simulink model "Speedgoat_FXLMS_ANC_model"  (R2022a)
settings: Solver=FixedStepDiscrete  StartTime=0.0  StopTime=inf  RelTol=1e-3
InitFcn:
  | L = 512;
  | FS = 8000;
  | %[noise,FS] = audioread('washing8kmod.wav');
StopFcn:
  | %postCallback;
undefined symbols (not defined in the file or in its folder): Ended, Single
libraries: speedgoatlib_IO104 x3, simulink x3, dspadpt3 x3, dspsrcs4 x2, slrealtimeobsoletelib x2, audiomeasurements x1
settings Model: SimulationMode=external  Creator=The MathWorks, Inc.  LastModifiedBy=Administrator
settings SolverCC: ConcurrentTasks=on  AlgebraicLoopSolver=TrustRegion  AutoInsertRateTranBlk=on  InsertRTBMode=Never (minimum delay)
settings DataIOCC: SaveFormat=StructureWithTime  ReturnWorkspaceOutputs=off
settings OptimizationCC: BlockReduction=off  OptimizeBlockIOStorage=off  BufferReuse=off  GlobalBufferReuse=off  ExpressionFolding=off  LocalBlockOutputs=off  OptimizeDataStoreBuffers=off  BusAssignmentInplaceUpdate=off
settings DebuggingCC: UnconnectedInputMsg=warning  UnconnectedOutputMsg=warning  UnconnectedLineMsg=warning  SFExecutionAtInitializationDiag=none  SFMachineParentedDataDiag=warning  ArithmeticOperatorsInVariantConditions=warning
settings HardwareCC: ProdBitPerPointer=32  ProdBitPerSizeT=32  ProdBitPerPtrDiffT=32  ProdLargestAtomicFloat=None  ProdWordSize=32  ProdLongLongMode=on  ProdHWDeviceType=Generic->32-bit x86 compatible
settings SFSimCC: SimUseLocalCustomCode=off  CustomCodeUndefinedFunction=UseInterfaceOnly
settings RTWCC: Description=Simulink Real-Time  SystemTargetFile=slrt.tlc  TLCOptions=-axPCMaxOverloads=10000 -axPCOverLoadLen=200  TemplateMakefile=slrt_default_tmf  RTWUseLocalCustomCode=off  RTWCompilerOptimization=on
settings CodeAppCC: StateflowObjectComments=on
settings SimulinkRealTimeCC: SupportVariableSizeSignals=on  OptimizeReductions=off  RL32LogTETModifier=off  RL32LogBufSizeModifier=100e6  RL32IRQSourceModifier=Auto (PCI only)  xPCConcurrentTasks=on

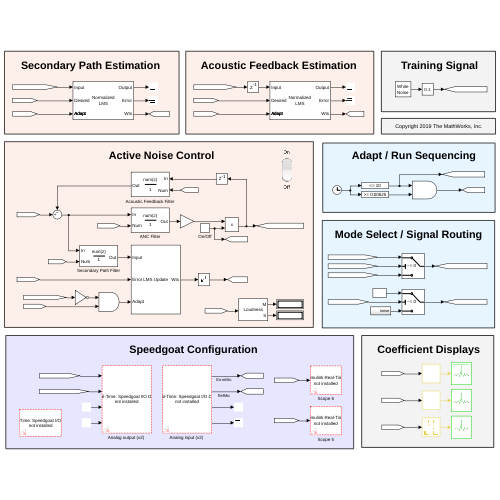
[thumbnail: Simulink's stored preview of the top-level diagram]
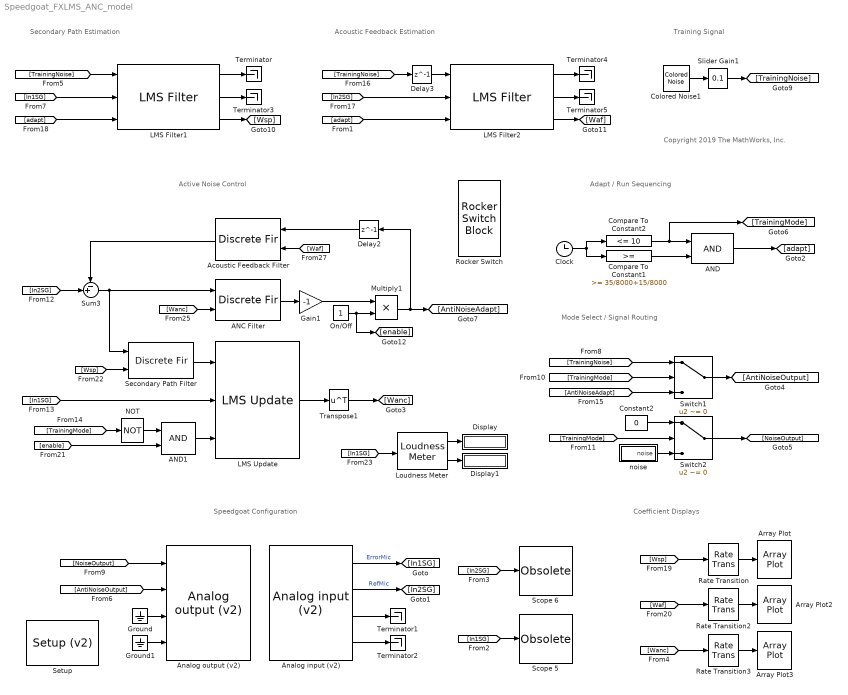
== system Speedgoat_FXLMS_ANC_model ==
  note: Copyright 2019 The MathWorks, Inc.
  note: Secondary Path Estimation
  note: Training Signal
  note: Mode Select / Signal Routing
  note: Speedgoat Configuration
  note: Acoustic Feedback Estimation
  note: Coefficient Displays
  note: Active Noise Control
  note: Adapt / Run Sequencing
  ANC Filter : DiscreteFir  CoefSource=Input port
      settings: InputPortMap=u0,u1
  AND : Logic  IconShape=distinctive  AllPortsSameDT=off  OutDataTypeStr=boolean
  AND1 : Logic  IconShape=distinctive  AllPortsSameDT=off  OutDataTypeStr=boolean
  Acoustic Feedback Filter : DiscreteFir  CoefSource=Input port
      settings: InputPortMap=u0,u1
  "Analog input (v2) " : speedgoatlib_IO104/Analog input (v2)   parModuleId=1  parTs=1/FS  parPciSlot=-1  parAdChannels=[1,2,3,4]  parAdChannelsSorted=[1,2,3,4]  parAdRange1=+-2.5V  parAdRange2=+-10V  parAdCoupling=Single-Ended  parAdFrameSize=1  parAdUseTrigger=on  parAdClockInitiator=Initiator  parAdSampleTime=1.250000000e-04  parTriggerInitiator=Initiator  parTriggerRate=1.250000000e-04
  "Analog output (v2) " : speedgoatlib_IO104/Analog output (v2)   parModuleId=1  parTs=-1  parPciSlot=-1  parDaChannels=[1,2,3,4]  parDaChannelsSorted=[1,2,3,4]  parDaInitValue=[0,0,0,0]  parDaReset=[1,1,1,1]  parDaRange=+-2.5V  parDaFrameSize=1  parDaUseTrigger=on  parDaClockInitiator=Initiator  parDaSampleTime=1.250000000e-04  parTriggerInitiator=Initiator  parTriggerRate=1.250000000e-04  parAdBlockPresent=1
  Array Plot : ArrayPlot  WindowPosition=[4.000000,380.000000,1912.000000,441.000000,]  ScopeFrameLocation=window  AxesScaling=Manual  YLimits=[-0.599393,0.958712]  DefaultConfigurationName=dsp.scopes.ArrayPlotBlockSpecification
  Array Plot2 : ArrayPlot  WindowPosition=[4 369 1913 463]  AxesScaling=Manual  YLimits=[-0.150075,0.145128]  DefaultConfigurationName=dsp.scopes.ArrayPlotBlockSpecification
  Array Plot3 : ArrayPlot  WindowPosition=[2702.000000,114.000000,976.000000,429.000000,]  ScopeFrameLocation=window  AxesScaling=Manual  YLimits=[-0.0225492,0.059565]  DefaultConfigurationName=dsp.scopes.ArrayPlotBlockSpecification
  Clock : Clock
  Colored Noise1 : dspsrcs4/Colored Noise  Color=white  InverseFrequencyPower=0.5  BoundedOutput=off  NumChannels=1  OutputDataType=double  SamplesPerFrame=1  SampleTime=1/FS  RandomStream=mt19937ar with seed  Seed=67  SimulateUsing=Code generation
      settings: SourceProductBaseCode=DS
  Compare To Constant1 : simulink/Logic and Bit Operations/Compare To Constant  relop=>=  const=35/8000+15/8000  OutDataTypeStr=boolean
  Compare To Constant2 : simulink/Logic and Bit Operations/Compare To Constant  relop=<=  const=10  OutDataTypeStr=boolean
  Constant2 : Constant  Value=0
  Delay2 : Delay  DelayLength=1
  Delay3 : Delay  DelayLength=1
  Display : Display
  Display1 : Display
  Gain1 : Gain  Gain=-1
  Ground : Ground
  Ground1 : Ground
  LMS Filter1 : dspadpt3/LMS Filter  Algo=Normalized LMS  L=L/2  stepflag=Dialog  mu=0.02  leakage=1.0  ic=0  Adapt=on  resetflag=None  weights=on  addnparflag=off  roundingMode=Floor  overflowMode=off
      settings: SourceProductBaseCode=DS
  LMS Filter2 : dspadpt3/LMS Filter  Algo=Normalized LMS  L=L/2  stepflag=Dialog  mu=0.02  leakage=1.0  ic=0  Adapt=on  resetflag=None  weights=on  addnparflag=off  roundingMode=Floor  overflowMode=off
      settings: SourceProductBaseCode=DS
  LMS Update : dspadpt3/LMS Update  Method=Normalized LMS  Length=L  NumFilters=1  StepSizeSource=Property  StepSize=0.002  LeakageFactor=1.0  InitialConditions=0  AdaptiveFilterMode=Tapped delay-line FIR filter  EnableAdaptInput=on  EnableResetInput=off  SimulateUsing=Code generation
      settings: SourceProductBaseCode=DS
  Loudness Meter : audiomeasurements/Loudness Meter  ChannelWeights=1  UseRelativeScale=on  TargetLoudness=-50.0  OutputTruePeak=off  InheritSampleRate=on  SampleRate=44100  SimulateUsing=Code generation
      settings: SourceProductBaseCode=AU
  Multiply1 : Product
  NOT : Logic  Operator=NOT  IconShape=distinctive  AllPortsSameDT=off  OutDataTypeStr=boolean
  On/Off : Constant
  Rate Transition : RateTransition  Deterministic=off  OutPortSampleTime=1/16
  Rate Transition2 : RateTransition  Deterministic=off  OutPortSampleTime=1/16
  Rate Transition3 : RateTransition  Deterministic=off  OutPortSampleTime=1/16
  Rocker Switch : RockerSwitchBlock  LabelPosition=Hide
      settings: Values={{'Off', 'On'}, [0 1]}
  Scope 5 : slrealtimeobsoletelib/Obsolete  ObsoleteBlock=slrtlib/Displays and Logging/Scope  ObsoleteParameters=|  NumInports=1  NumOutports=0
      | ContentPreviewEnabled:  off
      | scopeno:  2
      | scopetype:  Target
      | autostart:  on
      | viewmode:  Graphical redraw
      | formatstr:  '%15.6f'
      | grid:  on
      | ylimits:  2*[-1 1]
      | nosamples:  1e3
      | noprepostsamples:  0
      | interleave:  1
      | triggermode:  FreeRun
      | triggersignal:  1
      | trigsignalfromport:  off
      | triggerlevel:  0.0
      | triggerslope:  Either
      | triggerscope:  1
      | triggersample:  0
      | filename:  data.dat
      | mode:  Lazy
      | writesize:  512
      | autorestart:  off
      | dynamicfilemode:  off
      | maxwritefilesize:  512*1024^2
      settings: SourceProductBaseCode=XP
  Scope 6 : slrealtimeobsoletelib/Obsolete  ObsoleteBlock=slrtlib/Displays and Logging/Scope  ObsoleteParameters=|  NumInports=1  NumOutports=0
      | ContentPreviewEnabled:  off
      | scopeno:  1
      | scopetype:  Target
      | autostart:  on
      | viewmode:  Graphical redraw
      | formatstr:  '%15.6f'
      | grid:  on
      | ylimits:  2*[-1 1]
      | nosamples:  1e3
      | noprepostsamples:  0
      | interleave:  1
      | triggermode:  FreeRun
      | triggersignal:  1
      | trigsignalfromport:  off
      | triggerlevel:  0.0
      | triggerslope:  Either
      | triggerscope:  1
      | triggersample:  0
      | filename:  data.dat
      | mode:  Lazy
      | writesize:  512
      | autorestart:  off
      | dynamicfilemode:  off
      | maxwritefilesize:  512*1024^2
      settings: SourceProductBaseCode=XP
  Secondary Path Filter : DiscreteFir  CoefSource=Input port
      settings: InputPortMap=u0,u1
  Setup : speedgoatlib_IO104/Setup (v2)   parPciSlot=-1  parModuleId=1  parTriggerInitiator=Initiator  parTriggerRate=1/FS  parCalibrate=off  parAdChannels=[1:4]  parAdRange1=+-2.5V  parAdRange2=+-10V  parAdCoupling=Single-Ended  parAdUseTrigger=on  parAdFrameSize=1  parAdClockInitiator=Initiator  parAdSampleTime=1/FS  parDaChannels=[1:4]  parDaChannelsSorted=0  parDaInitValue=[0]  parDaReset=[1]  parDaRange=+-2.5V  parDaUseTrigger=on  parDaFrameSize=1  parDaClockInitiator=Initiator  parDaSampleTime=1/FS  parDioByte0Dir=Outputs  parDioByte1Dir=Inputs  parDoChannels=0  parDoInitValues=[0]  parDoReset=[1]  parDiChannels=0
  Slider Gain1 : simulink/Math Operations/Slider Gain  gain=0.1  low=0  high=1
  Sum3 : Sum  Inputs=-+|
  Switch1 : Switch  Criteria=u2 ~= 0  Threshold=5  SaturateOnIntegerOverflow=off  InputSameDT=off
  Switch2 : Switch  Criteria=u2 ~= 0  Threshold=5  SaturateOnIntegerOverflow=off  InputSameDT=off
  Terminator{,1..5} (6 alike) : Terminator
  Transpose1 : Math  Operator=transpose  SignedPower=on
  noise : Subsystem
  wires:
  "Analog input (v2) "/4 -> Terminator2/1
  "Analog input (v2) "/3 -> Terminator1/1
  Ground/1 -> "Analog output (v2) "/3
  Ground1/1 -> "Analog output (v2) "/4
  "Analog input (v2) "/1 -> [In1SG]  "ErrorMic"
  [In1SG] -> Scope 5/1
  [In2SG] -> Scope 6/1
  "Analog input (v2) "/2 -> [In2SG]  "RefMic"
  [NoiseOutput] -> "Analog output (v2) "/1
  [AntiNoiseOutput] -> "Analog output (v2) "/2
  Colored Noise1/1 -> Slider Gain1/1
  Slider Gain1/1 -> [TrainingNoise]
  Switch1/1 -> [AntiNoiseOutput]
  [TrainingNoise] -> Switch1/1
  Constant2/1 -> Switch2/1
  Switch2/1 -> [NoiseOutput]
  [TrainingMode] -> Switch1/2
  [TrainingMode] -> Switch2/2
  [TrainingMode] -> NOT/1
  [AntiNoiseAdapt] -> Switch1/3
  NOT/1 -> AND1/1
  AND1/1 -> LMS Update/3
  Multiply1/1 -> Delay2/1, [AntiNoiseAdapt]
  noise/1(noise) -> Switch2/3
  ANC Filter/1 -> Gain1/1
  [Wsp] -> Secondary Path Filter/2
  Rate Transition/1 -> Array Plot/1
  [In1SG] -> LMS Filter1/2
  [TrainingNoise] -> LMS Filter1/1
  Rate Transition2/1 -> Array Plot2/1
  [TrainingNoise] -> Delay3/1
  [In2SG] -> LMS Filter2/2
  LMS Filter2/1 -> Terminator4/1
  LMS Filter2/2 -> Terminator5/1
  LMS Filter2/3 -> [Waf]
  LMS Update/1 -> Transpose1/1
  [In2SG] -> Sum3/2
  Sum3/1 -> ANC Filter/1, Secondary Path Filter/1
  Secondary Path Filter/1 -> LMS Update/1
  [In1SG] -> LMS Update/2
  [adapt] -> LMS Filter2/3
  LMS Filter1/3 -> [Wsp]
  LMS Filter1/2 -> Terminator3/1
  LMS Filter1/1 -> Terminator/1
  Rate Transition3/1 -> Array Plot3/1
  [enable] -> AND1/2
  Gain1/1 -> Multiply1/1
  On/Off/1 -> Multiply1/2, [enable]
  Transpose1/1 -> [Wanc]
  [Wanc] -> ANC Filter/2
  Acoustic Feedback Filter/1 -> Sum3/1
  [Waf] -> Acoustic Feedback Filter/2
  Compare To Constant1/1 -> AND/2
  AND/1 -> [adapt]
  Compare To Constant2/1 -> [TrainingMode], AND/1
  Clock/1 -> Compare To Constant2/1, Compare To Constant1/1
  [adapt] -> LMS Filter1/3
  Delay2/1 -> Acoustic Feedback Filter/1
  Delay3/1 -> LMS Filter2/1
  [Wsp] -> Rate Transition/1
  [Waf] -> Rate Transition2/1
  [Wanc] -> Rate Transition3/1
  [In1SG] -> Loudness Meter/1
  Loudness Meter/1 -> Display/1
  Loudness Meter/2 -> Display1/1

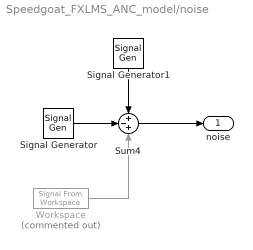
== system Speedgoat_FXLMS_ANC_model/noise ==
  Signal Generator : SignalGenerator  Amplitude=.2  Frequency=150
  Signal Generator1 : SignalGenerator  Amplitude=.15  Frequency=225
  Sum4 : Sum  Inputs=+-+
  Workspace : dspsrcs4/Signal From Workspace  Commented=on  X=noise  Ts=1/FS  nsamps=1  OutputAfterFinalValue=Cyclic repetition  ignoreOrWarnInputAndFrameLengths=off  OutputFrames=off
  noise : Outport  VectorParamsAs1DForOutWhenUnconnected=off
  wires:
  Signal Generator/1 -> Sum4/2
  Signal Generator1/1 -> Sum4/1
  Sum4/1 -> noise/1
  Workspace/1 -> Sum4/3
